simulink model "pwm"  (R2023b)
settings: Solver=VariableStepAuto  StartTime=0.0  StopTime=2  RelTol=1e-3
libraries: simulink x7, spsMosfetLib x6, spsTriangleGeneratorLib x4, spsSeriesRLCBranchLib x2, spsDCVoltageSourceLib x1, spsDiodeLib x1, spsVoltageMeasurementLib x1, sps_lib x1
settings Model: Creator=NIT  LastModifiedBy=mluser
settings SolverCC: AlgebraicLoopSolver=TrustRegion
settings DataIOCC: ReturnWorkspaceOutputs=off
settings DebuggingCC: UnconnectedInputMsg=warning  UnconnectedOutputMsg=warning  UnconnectedLineMsg=warning  ArithmeticOperatorsInVariantConditions=warning
settings ModelReferenceCC: EnableRefExpFcnMdlSchedulingChecks=on
settings SFSimCC: SimUseLocalCustomCode=off  CustomCodeUndefinedFunction=UseInterfaceOnly
settings RTWCC: RTWUseLocalCustomCode=off

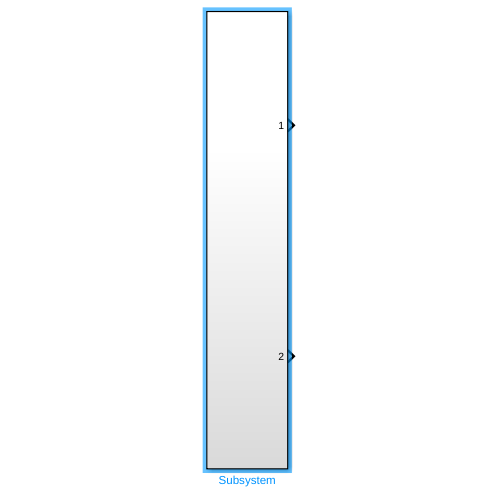
[thumbnail: Simulink's stored preview of the top-level diagram]
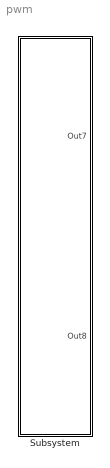
== system pwm ==
  Subsystem : Subsystem

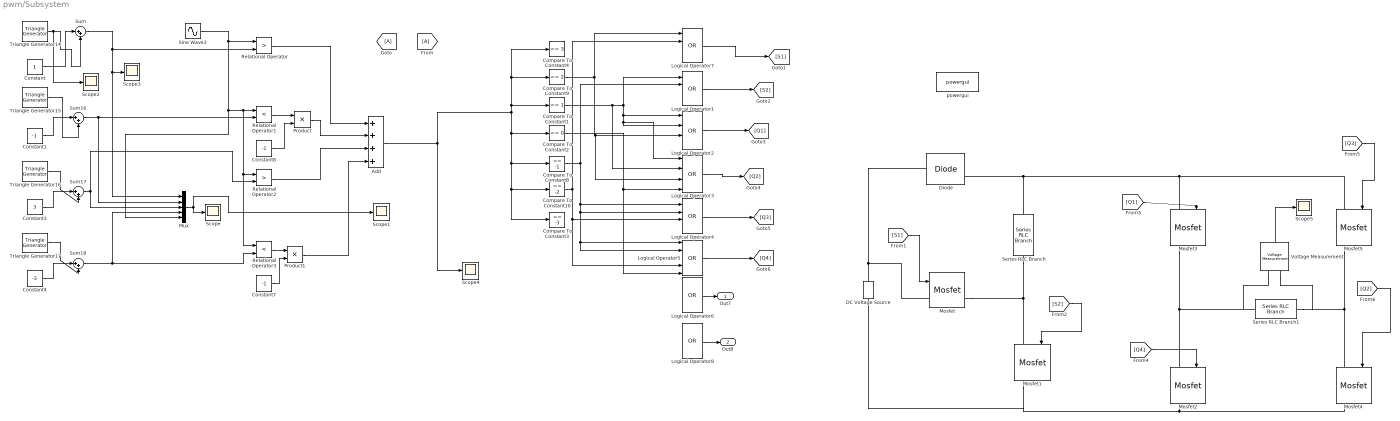
== system pwm/Subsystem ==
  Add : Sum  Inputs=++++
  Compare To Constant1 : simulink/Logic and Bit Operations/Compare To Constant  relop===  const=1  OutDataTypeStr=boolean
  Compare To Constant10 : simulink/Logic and Bit Operations/Compare To Constant  relop===  const=-2  OutDataTypeStr=boolean
  Compare To Constant2 : simulink/Logic and Bit Operations/Compare To Constant  relop===  const=0  OutDataTypeStr=boolean
  Compare To Constant3 : simulink/Logic and Bit Operations/Compare To Constant  relop===  const=-3  OutDataTypeStr=boolean
  Compare To Constant4 : simulink/Logic and Bit Operations/Compare To Constant  relop===  const=3  OutDataTypeStr=boolean
  Compare To Constant8 : simulink/Logic and Bit Operations/Compare To Constant  relop===  const=-1  OutDataTypeStr=boolean
  Compare To Constant9 : simulink/Logic and Bit Operations/Compare To Constant  relop===  const=2  OutDataTypeStr=boolean
  Constant : Constant
  Constant1 : Constant  Value=-1
  Constant3 : Constant  Value=3
  Constant4 : Constant  Value=-3
  Constant7 : Constant  Value=-1
  Constant8 : Constant  Value=-1
  DC Voltage Source : spsDCVoltageSourceLib/DC Voltage Source  Amplitude=160  Measurements=None
  Diode : spsDiodeLib/Diode  Ron=0.001  Lon=0  Vf=0.8  IC=0  UseSnubber=0  Rs=500  Cs=250e-9  Measurements=on
  From : From
  Goto : Goto
  Logical Operator{1..4,6..8} (7 alike) : Logic  Operator=OR  Inputs=4  AllPortsSameDT=off  OutDataTypeStr=boolean
  Logical Operator5 : Logic  Operator=OR  Inputs=5  AllPortsSameDT=off  OutDataTypeStr=boolean
  Mosfet{,1..5} (6 alike) : spsMosfetLib/Mosfet  Ron=0.1  Lon=0  Rd=0.01  Vfd=0  IC=0  Rs=1e5  Cs=inf  Measurements=on
  Mux : Mux  Inputs=5
  Product : Product
  Product1 : Product
  Relational Operator : RelationalOperator  Operator=>  OutDataTypeStr=boolean  InputSameDT=off
  Relational Operator1 : RelationalOperator  Operator=<  OutDataTypeStr=boolean  InputSameDT=off
  Relational Operator2 : RelationalOperator  Operator=>  OutDataTypeStr=boolean  InputSameDT=off
  Relational Operator3 : RelationalOperator  Operator=<  OutDataTypeStr=boolean  InputSameDT=off
  Scope{,1..5} (6 alike) : Scope
  Series RLC Branch : spsSeriesRLCBranchLib/Series RLC Branch  LConnTagsString=__new0  RConnTagsString=__new0  BranchType=C  Resistance=1  Inductance=1e-3  SetiL0=off  InitialCurrent=0  Capacitance=1/1000  Setx0=off  InitialVoltage=0  Measurements=None
  Series RLC Branch1 : spsSeriesRLCBranchLib/Series RLC Branch  LConnTagsString=__new0  RConnTagsString=__new0  BranchType=R  Resistance=10  Inductance=1e-3  SetiL0=off  InitialCurrent=0  Capacitance=1e-6  Setx0=off  InitialVoltage=0  Measurements=None
  Sine Wave3 : Sin  Amplitude=4  Frequency=2*pi*50  SampleTime=0
  Sum{,16..18} (4 alike) : Sum  Inputs=|++
  Triangle Generator14 : spsTriangleGeneratorLib/Triangle Generator  Freq=100  Phase=180  Ts=0
  Triangle Generator15 : spsTriangleGeneratorLib/Triangle Generator  Freq=100  Phase=0  Ts=0
  Triangle Generator16 : spsTriangleGeneratorLib/Triangle Generator  Freq=100  Phase=180  Ts=0
  Triangle Generator17 : spsTriangleGeneratorLib/Triangle Generator  Freq=100  Phase=0  Ts=0
  Voltage Measurement : spsVoltageMeasurementLib/Voltage Measurement  PhasorSimulation=off  OutputType=Complex  PSBequivalent=0
  powergui : sps_lib/powergui  Priority=1  SimulationMode=Continuous  SampleTime=50e-6  frequency=60  Iterations=50  frequencyindice=0  Pbase=100e6  ErrMax=1e-4  UnitsV=kV  UnitsW=MW  buscounter=0  FunctionMessages=off  echomessages=off  EnableUseOfTLC=off  CurrentSourceSwitches=off  DisableSnubberDevices=off  DisableRonSwitches=off  DisableVfSwitches=off  DisplayEquations=off  AutomaticDiscreteSolvers=off  SolverType=Tustin/Backward Euler (TBE)  Interpol=off  ExternalGateDelay=off  methode=off  Ts=100  x0status=blocks  SPID=on  SwTol=0  HookPort=off  NonlinearTolerance=1e-4  nMaxIteration=100  ContinueOnMaxIteration=off  RestoreLinks=warning  ResistiveCurrentMeasurement=off  Frange=[0:2:500]  Ylog=off  Xlog=on  ShowGrid=off  save=off  variable=ZData  structure=0  ZoomFFT=off  StartTime=0.0  cycles=1  DisplayStyle=1  fundamental=60  FreqAxis=off  MaxFrequency=1000  frequencyindicesteady=1  RmsSteady=1  display=off
  Out7 : Outport  VectorParamsAs1DForOutWhenUnconnected=off
  Out8 : Outport  Port=2  VectorParamsAs1DForOutWhenUnconnected=off
  wires:
  Relational Operator2/1 -> Add/3
  Product1/1 -> Add/4
  Product/1 -> Add/2
  Constant8/1 -> Product/2
  Sum16/1 -> Mux/2, Relational Operator1/2
  Relational Operator/1 -> Add/1
  Relational Operator3/1 -> Product1/1
  Constant7/1 -> Product1/2
  Mux/1 -> Scope/1, Scope1/1
  Relational Operator1/1 -> Product/1
  Triangle Generator17/1 -> Sum18/2
  Constant/1 -> Sum/1
  Triangle Generator15/1 -> Sum16/2
  Sum18/1 -> Mux/4, Relational Operator3/2
  Constant1/1 -> Sum16/1
  Constant4/1 -> Sum18/1
  Constant3/1 -> Sum17/1
  Triangle Generator16/1 -> Sum17/2
  Sum17/1 -> Relational Operator2/2, Mux/3
  Sum/1 -> Scope3/1, Mux/1, Relational Operator/2
  Triangle Generator14/1 -> Scope2/1, Sum/2
  Sine Wave3/1 -> Mux/5, Relational Operator3/1, Relational Operator2/1, Relational Operator1/1, Relational Operator/1
  Add/1 -> Scope4/1, Compare To Constant2/1, Compare To Constant3/1, Compare To Constant10/1, Compare To Constant8/1, Compare To Constant4/1, Compare To Constant9/1, Compare To Constant1/1
  Logical Operator6/1 -> Out7/1
  Logical Operator8/1 -> Out8/1
  Voltage Measurement/1 -> Scope5/1
  [S1] -> Mosfet/1
  [Q1] -> Mosfet3/1
  [S2] -> Mosfet1/1
  [Q4] -> Mosfet2/1
  [Q2] -> Mosfet4/1
  [Q3] -> Mosfet5/1
  Logical Operator7/1 -> [S1]
  Logical Operator1/1 -> [S2]
  Logical Operator2/1 -> [Q1]
  Logical Operator3/1 -> [Q2]
  Logical Operator4/1 -> [Q3]
  Logical Operator5/1 -> [Q4]
  Compare To Constant2/1 -> Logical Operator3/4, Logical Operator5/5
  Compare To Constant1/1 -> Logical Operator3/2, Logical Operator2/2, Logical Operator3/1, Logical Operator2/1, Logical Operator1/1
  Compare To Constant9/1 -> Logical Operator7/1, Logical Operator3/3, Logical Operator2/3
  Compare To Constant8/1 -> Logical Operator5/2, Logical Operator5/1, Logical Operator4/2, Logical Operator4/1, Logical Operator1/2
  Compare To Constant10/1 -> Logical Operator4/3, Logical Operator5/4, Logical Operator7/2
  connections:
  Mosfet3/RConn1 -- Voltage Measurement/LConn1 -- Series RLC Branch1/LConn1 -- Mosfet2/LConn1
  Mosfet5/RConn1 -- Voltage Measurement/LConn2 -- Series RLC Branch1/RConn1 -- Mosfet4/LConn1
  Mosfet3/LConn1 -- Series RLC Branch/LConn1 -- Diode/RConn1 -- Mosfet5/LConn1
  Mosfet4/RConn1 -- DC Voltage Source/LConn1 -- Mosfet1/RConn1 -- Mosfet2/RConn1
  Series RLC Branch/RConn1 -- Mosfet/RConn1 -- Mosfet1/LConn1
  DC Voltage Source/RConn1 -- Diode/LConn1 -- Mosfet/LConn1
